simulink model "MagLevCtrl"  (R2025b)
settings: Solver=FixedStepDiscrete  StartTime=0.0  StopTime=Inf  FixedStep=Ts  RelTol=1e-3  EnableMultiTasking=on
undefined symbols (not defined in the file or in its folder): ctrl, DiscIntNeverNeededParam, enable, sens, X, Y
libraries: MagLevTbx_BaseLib x10, simulink x4
settings Model: ExtModeTrigDuration=2  Creator=riccardo  LastModifiedBy=riccardo
settings SolverCC: AutoInsertRateTranBlk=on
settings DataIOCC: ReturnWorkspaceOutputs=off
settings OptimizationCC: StrengthReduction=on  PassReuseOutputArgsAs=Individual arguments  ZeroExternalMemoryAtStartup=off  ZeroInternalMemoryAtStartup=off  MaxStackSize=64  OptimizeBlockOrder=speed  OptimizationPriority=Speed  OptimizationCustomize=off  MultiThreadedLoops=on  AutoScheduleForLoops=on  EfficientTunableParamExpr=on
settings DebuggingCC: ParameterTunabilityLossMsg=error
settings HardwareCC: ProdBitPerPointer=32.0  ProdBitPerSizeT=32.0  ProdBitPerPtrDiffT=32.0  ProdLargestAtomicInteger=Long  ProdLargestAtomicFloat=Double  ProdWordSize=32.0  ProdHWDeviceType=ARM Compatible->ARM Cortex
settings SFSimCC: MATLABDynamicMemAlloc=off
settings RTWCC: SystemTargetFile=ert.tlc  HardwareBoard=Teensy 4.1 (Arduino Compatible)  TemplateMakefile=ert_default_tmf  Toolchain=Arduino ARM M7  BuildConfiguration=Faster Runs  Description=Embedded Coder
settings CodeAppCC: ForceParamTrailComments=on  IgnoreCustomStorageClasses=off  OperatorAnnotations=on  SimulinkDataObjDesc=on  SFDataObjDesc=on  InsertBlockDesc=on
settings ERTTargetCC: ExtModeTransport=3.0  ExtModeStaticAlloc=on  ExtModeAutomaticAllocSize=off  ExtModeStaticAllocSize=65536.0  ExtModeMexFile=ext_xcp  ExtModeIntrfLevel=Level2 - Open  InlinedParameterPlacement=Hierarchical  RootIOFormat=Structure reference  TargetLangStandard=C99 (ISO)  SupportContinuousTime=on  SupportVariableSizeSignals=on

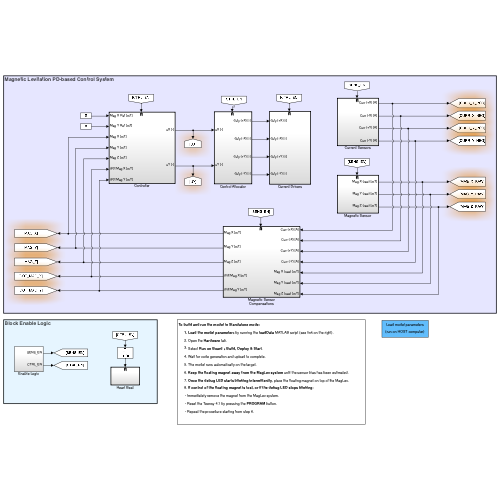
[thumbnail: Simulink's stored preview of the top-level diagram]
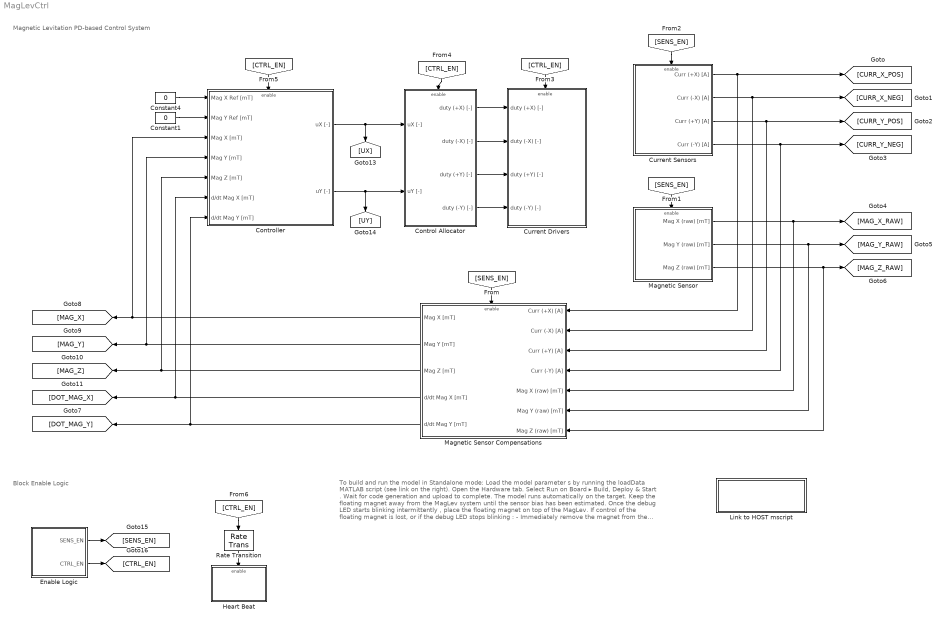
== system MagLevCtrl ==
  note: Block Enable Logic
  note: Magnetic Levitation PD-based Control System
  note: To build and run the model in Standalone mode:
      | Load the model parameter s by running the loadData MATLAB script (see link on the right).
      | Open the Hardware tab.
      | Select Run on Board ▸ Build, Deploy & Start .
      | Wait for code generation and upload to complete.
      | The model runs automatically on the target.
      | Keep the floating magnet away from the MagLev system until the sensor bias has been estimated.
      | Once the debug LED starts blinking intermittently , place the floating magnet on top of the MagLev.
      | If control of the floating magnet is lost, or if the debug LED stops blinking :
      | - Immediately remove the magnet from the MagLev system.
      | - Reset the Teensy 4.1 by pressing the PROGRAM button.
      | - Repeat the procedure starting from step 6.
  Constant1 : Constant  Value=0  OutDataTypeStr=single  SampleTime=ctrl.Ts
  Constant4 : Constant  Value=0  OutDataTypeStr=single  SampleTime=ctrl.Ts
  Control Allocator : Subsystem
  Controller : Subsystem
  Current Drivers : Subsystem
  Current Sensors : Subsystem
  Enable Logic : Subsystem
  Heart Beat : Subsystem
  Link to HOST mscript : Subsystem
      settings: OpenFcn=|
      | %  get toolbox base dir
      | info = MagLevTbx_Info();
      | 
      | %  path to HOST matlab script
      | mscriptpath = fullfile( ...
      | info.rootDir, ...
      | 'Examples', ...
      | 'Ctrl_Test', ...
      | 'Standalone', ...
      | 'loadData'  );
      | 
      | %  open script
      | edit( mscriptpath );
      | 
      | %  clear temp vars
      | clear info mscriptpath;
      mask Display:
      | disp(['Load model parameters\n\n' ...
      |     '(run on HOST computer)'])
  Magnetic Sensor : Subsystem
  Magnetic Sensor Compensations : Subsystem
  Rate Transition : RateTransition  OutPortSampleTime=enable.heartBeat_Ts
  wires:
  Current Sensors/1(Curr (+X) [A]) -> Magnetic Sensor Compensations/1(Curr (+X) [A]), [CURR_X_POS]
  Current Sensors/2(Curr (-X) [A]) -> Magnetic Sensor Compensations/2(Curr (-X) [A]), [CURR_X_NEG]
  Current Sensors/3(Curr (+Y) [A]) -> Magnetic Sensor Compensations/3(Curr (+Y) [A]), [CURR_Y_POS]
  Current Sensors/4(Curr (-Y) [A]) -> Magnetic Sensor Compensations/4(Curr (-Y) [A]), [CURR_Y_NEG]
  Magnetic Sensor/1(Mag X (raw) [mT]) -> Magnetic Sensor Compensations/5(Mag X (raw) [mT]), [MAG_X_RAW]
  Magnetic Sensor/2(Mag Y (raw) [mT]) -> Magnetic Sensor Compensations/6(Mag Y (raw) [mT]), [MAG_Y_RAW]
  Magnetic Sensor/3(Mag Z (raw) [mT]) -> Magnetic Sensor Compensations/7(Mag Z (raw) [mT]), [MAG_Z_RAW]
  Control Allocator/1(duty (+X) [-]) -> Current Drivers/1(duty (+X) [-])
  Control Allocator/2(duty (-X) [-]) -> Current Drivers/2(duty (-X) [-])
  Control Allocator/3(duty (+Y) [-]) -> Current Drivers/3(duty (+Y) [-])
  Control Allocator/4(duty (-Y) [-]) -> Current Drivers/4(duty (-Y) [-])
  Magnetic Sensor Compensations/2(Mag Y [mT]) -> [MAG_Y], Controller/4(Mag Y [mT])
  Magnetic Sensor Compensations/1(Mag X [mT]) -> [MAG_X], Controller/3(Mag X [mT])
  Constant4/1 -> Controller/1(Mag X Ref [mT])
  Constant1/1 -> Controller/2(Mag Y Ref [mT])
  Magnetic Sensor Compensations/4(d/dt Mag X [mT]) -> [DOT_MAG_X], Controller/6(d/dt Mag X [mT])
  Magnetic Sensor Compensations/5(d/dt Mag Y [mT]) -> [DOT_MAG_Y], Controller/7(d/dt Mag Y [mT])
  Magnetic Sensor Compensations/3(Mag Z [mT]) -> [MAG_Z], Controller/5(Mag Z [mT])
  [SENS_EN] -> Magnetic Sensor Compensations/Enable
  [SENS_EN] -> Magnetic Sensor/Enable
  [CTRL_EN] -> Control Allocator/Enable
  [CTRL_EN] -> Controller/Enable
  Enable Logic/1(SENS_EN) -> [SENS_EN]
  [SENS_EN] -> Current Sensors/Enable
  Enable Logic/2(CTRL_EN) -> [CTRL_EN]
  [CTRL_EN] -> Current Drivers/Enable
  Controller/1(uX [-]) -> Control Allocator/1(uX [-]), [UX]
  Controller/2(uY [-]) -> Control Allocator/2(uY [-]), [UY]
  [CTRL_EN] -> Rate Transition/1
  Rate Transition/1 -> Heart Beat/Enable

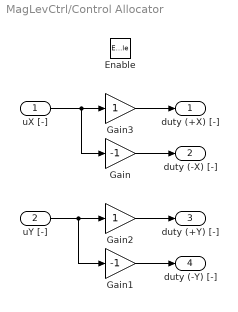
== system MagLevCtrl/Control Allocator ==
  uX [-] : Inport
  uY [-] : Inport  Port=2
  Enable : EnablePort
  Gain : Gain  Gain=-1
  Gain1 : Gain  Gain=-1
  Gain2 : Gain
  Gain3 : Gain
  duty (+X) [-] : Outport  OutputWhenDisabled=reset  InitialOutput=0
  duty (-X) [-] : Outport  Port=2  OutputWhenDisabled=reset  InitialOutput=0
  duty (+Y) [-] : Outport  Port=3  OutputWhenDisabled=reset  InitialOutput=0
  duty (-Y) [-] : Outport  Port=4  OutputWhenDisabled=reset  InitialOutput=0
  wires:
  uX [-]/1 -> Gain3/1, Gain/1
  Gain/1 -> duty (-X) [-]/1
  Gain1/1 -> duty (-Y) [-]/1
  uY [-]/1 -> Gain2/1, Gain1/1
  Gain2/1 -> duty (+Y) [-]/1
  Gain3/1 -> duty (+X) [-]/1

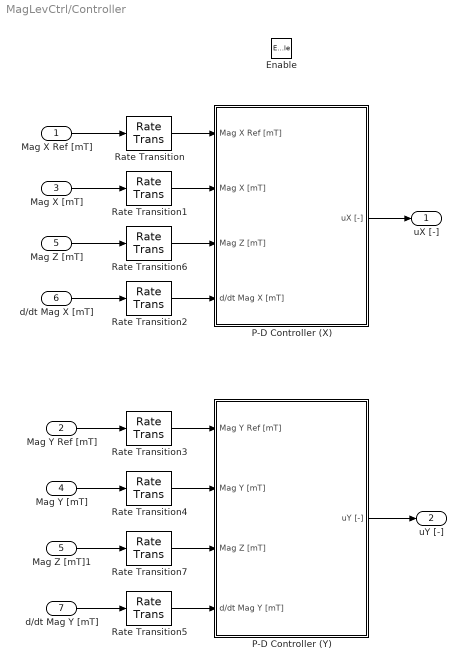
== system MagLevCtrl/Controller ==
  Mag X Ref [mT] : Inport
  Mag Y Ref [mT] : Inport  Port=2
  Mag X [mT] : Inport  Port=3
  Mag Y [mT] : Inport  Port=4
  Mag Z [mT] : Inport  Port=5
  d/dt Mag X [mT] : Inport  Port=6
  d/dt Mag Y [mT] : Inport  Port=7
  Enable : EnablePort
  Mag Z [mT]1 : InportShadow  Port=5
  P-D Controller (X) : Subsystem
  P-D Controller (Y) : Subsystem
  Rate Transition{,1..7} (8 alike) : RateTransition  OutPortSampleTime=ctrl.Ts
  uX [-] : Outport  OutputWhenDisabled=reset  InitialOutput=0
  uY [-] : Outport  Port=2  OutputWhenDisabled=reset  InitialOutput=0
  wires:
  d/dt Mag Y [mT]/1 -> Rate Transition5/1
  P-D Controller (Y)/1(uY [-]) -> uY [-]/1
  Mag Y Ref [mT]/1 -> Rate Transition3/1
  Mag X Ref [mT]/1 -> Rate Transition/1
  P-D Controller (X)/1(uX [-]) -> uX [-]/1
  Mag X [mT]/1 -> Rate Transition1/1
  Mag Y [mT]/1 -> Rate Transition4/1
  d/dt Mag X [mT]/1 -> Rate Transition2/1
  Rate Transition/1 -> P-D Controller (X)/1(Mag X Ref [mT])
  Rate Transition1/1 -> P-D Controller (X)/2(Mag X [mT])
  Rate Transition2/1 -> P-D Controller (X)/4(d/dt Mag X [mT])
  Rate Transition3/1 -> P-D Controller (Y)/1(Mag Y Ref [mT])
  Rate Transition4/1 -> P-D Controller (Y)/2(Mag Y [mT])
  Rate Transition5/1 -> P-D Controller (Y)/4(d/dt Mag Y [mT])
  Mag Z [mT]/1 -> Rate Transition6/1
  Rate Transition6/1 -> P-D Controller (X)/3(Mag Z [mT])
  Mag Z [mT]1/1 -> Rate Transition7/1
  Rate Transition7/1 -> P-D Controller (Y)/3(Mag Z [mT])

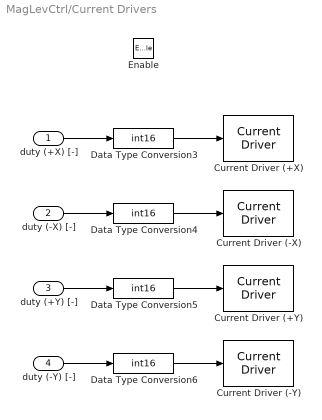
== system MagLevCtrl/Current Drivers ==
  duty (+X) [-] : Inport
  duty (-X) [-] : Inport  Port=2
  duty (+Y) [-] : Inport  Port=3
  duty (-Y) [-] : Inport  Port=4
  Enable : EnablePort
  Current Driver (+X) : MagLevTbx_BaseLib/Outputs/Current Driver  driverId=+X  sampleTime=ctrl.Ts  showEnablePort=off
      settings: SourceProductName=MagLev Toolbox
  Current Driver (+Y) : MagLevTbx_BaseLib/Outputs/Current Driver  driverId=+Y  sampleTime=ctrl.Ts  showEnablePort=off
      settings: SourceProductName=MagLev Toolbox
  Current Driver (-X) : MagLevTbx_BaseLib/Outputs/Current Driver  driverId=-X  sampleTime=ctrl.Ts  showEnablePort=off
      settings: SourceProductName=MagLev Toolbox
  Current Driver (-Y) : MagLevTbx_BaseLib/Outputs/Current Driver  driverId=-Y  sampleTime=ctrl.Ts  showEnablePort=off
      settings: SourceProductName=MagLev Toolbox
  Data Type Conversion{3..6} (4 alike) : DataTypeConversion  OutDataTypeStr=int16  SaturateOnIntegerOverflow=off  RndMeth=Floor
  wires:
  duty (+Y) [-]/1 -> Data Type Conversion5/1
  Data Type Conversion5/1 -> Current Driver (+Y)/1
  Data Type Conversion6/1 -> Current Driver (-Y)/1
  duty (-Y) [-]/1 -> Data Type Conversion6/1
  Data Type Conversion4/1 -> Current Driver (-X)/1
  duty (+X) [-]/1 -> Data Type Conversion3/1
  duty (-X) [-]/1 -> Data Type Conversion4/1
  Data Type Conversion3/1 -> Current Driver (+X)/1

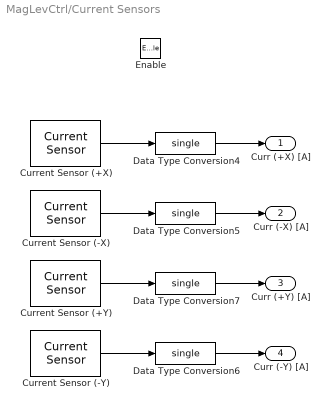
== system MagLevCtrl/Current Sensors ==
  Enable : EnablePort
  Current Sensor (+X) : MagLevTbx_BaseLib/Inputs/Current Sensor  sensorId=+X  sampleTime=sens.Ts  showEnablePort=off
      settings: SourceProductName=MagLev Toolbox
  Current Sensor (+Y) : MagLevTbx_BaseLib/Inputs/Current Sensor  sensorId=+Y  sampleTime=sens.Ts  showEnablePort=off
      settings: SourceProductName=MagLev Toolbox
  Current Sensor (-X) : MagLevTbx_BaseLib/Inputs/Current Sensor  sensorId=-X  sampleTime=sens.Ts  showEnablePort=off
      settings: SourceProductName=MagLev Toolbox
  Current Sensor (-Y) : MagLevTbx_BaseLib/Inputs/Current Sensor  sensorId=-Y  sampleTime=sens.Ts  showEnablePort=off
      settings: SourceProductName=MagLev Toolbox
  Data Type Conversion{4..7} (4 alike) : DataTypeConversion  OutDataTypeStr=single  SaturateOnIntegerOverflow=off  RndMeth=Floor
  Curr (+X) [A] : Outport
  Curr (-X) [A] : Outport  Port=2
  Curr (+Y) [A] : Outport  Port=3
  Curr (-Y) [A] : Outport  Port=4
  wires:
  Data Type Conversion5/1 -> Curr (-X) [A]/1
  Data Type Conversion4/1 -> Curr (+X) [A]/1
  Data Type Conversion7/1 -> Curr (+Y) [A]/1
  Data Type Conversion6/1 -> Curr (-Y) [A]/1
  Current Sensor (+X)/1 -> Data Type Conversion4/1
  Current Sensor (-X)/1 -> Data Type Conversion5/1
  Current Sensor (+Y)/1 -> Data Type Conversion7/1
  Current Sensor (-Y)/1 -> Data Type Conversion6/1

== system MagLevCtrl/Enable Logic ==
  Clock : Clock
  Interval Test : simulink/Logic and Bit Operations/Interval Test  IntervalClosedRight=on  uplimit=enable.ctrlTurnOffTime  IntervalClosedLeft=on  lowlimit=enable.ctrlTurnOnTime  OutDataTypeStr=boolean
  Interval Test1 : simulink/Logic and Bit Operations/Interval Test  IntervalClosedRight=on  uplimit=enable.sensTurnOffTime  IntervalClosedLeft=on  lowlimit=enable.sensTurnOnTime  OutDataTypeStr=boolean
  Rate Transition : RateTransition  OutPortSampleTime=enable.Ts
  Rate Transition1 : RateTransition  OutPortSampleTime=enable.Ts
  SENS_EN : Outport
  CTRL_EN : Outport  Port=2
  wires:
  Interval Test/1 -> Rate Transition/1
  Rate Transition/1 -> CTRL_EN/1
  Clock/1 -> Interval Test/1, Interval Test1/1
  Interval Test1/1 -> Rate Transition1/1
  Rate Transition1/1 -> SENS_EN/1

== system MagLevCtrl/Heart Beat ==
  Enable : EnablePort
  Data Type Conversion3 : DataTypeConversion  OutDataTypeStr=boolean  SaturateOnIntegerOverflow=off  RndMeth=Floor
  Repeating Sequence Stair : simulink/Sources/Repeating Sequence Stair  OutValues=[1 0].'  tsamp=enable.heartBeat_Ts  OutMin=[]  OutMax=[]  OutDataTypeStr=double  OutputDataTypeScalingMode=double  OutDataType=fixdt(0,8)  ConRadixGroup=Best Precision: Vector-wise  OutScaling=2^-12
  User LED : MagLevTbx_BaseLib/Outputs/User LED  sampleTime=-1  showEnablePort=off
      settings: SourceProductName=MagLev Toolbox
  wires:
  Repeating Sequence Stair/1 -> Data Type Conversion3/1
  Data Type Conversion3/1 -> User LED/1

== system MagLevCtrl/Link to HOST mscript ==

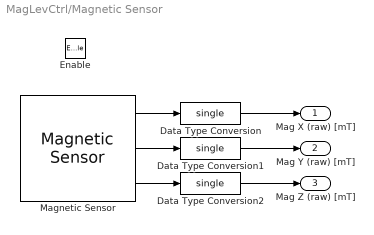
== system MagLevCtrl/Magnetic Sensor ==
  Enable : EnablePort
  Data Type Conversion : DataTypeConversion  OutDataTypeStr=single  SaturateOnIntegerOverflow=off  RndMeth=Floor
  Data Type Conversion1 : DataTypeConversion  OutDataTypeStr=single  SaturateOnIntegerOverflow=off  RndMeth=Floor
  Data Type Conversion2 : DataTypeConversion  OutDataTypeStr=single  SaturateOnIntegerOverflow=off  RndMeth=Floor
  Magnetic Sensor : MagLevTbx_BaseLib/Inputs/Magnetic Sensor  sensorId=Sensor 7  sampleTime=sens.Ts  showEnablePort=off
      settings: SourceProductName=MagLev Toolbox
  Mag X (raw) [mT] : Outport
  Mag Y (raw) [mT] : Outport  Port=2
  Mag Z (raw) [mT] : Outport  Port=3
  wires:
  Data Type Conversion1/1 -> Mag Y (raw) [mT]/1
  Data Type Conversion2/1 -> Mag Z (raw) [mT]/1
  Magnetic Sensor/2 -> Data Type Conversion1/1
  Data Type Conversion/1 -> Mag X (raw) [mT]/1
  Magnetic Sensor/1 -> Data Type Conversion/1
  Magnetic Sensor/3 -> Data Type Conversion2/1

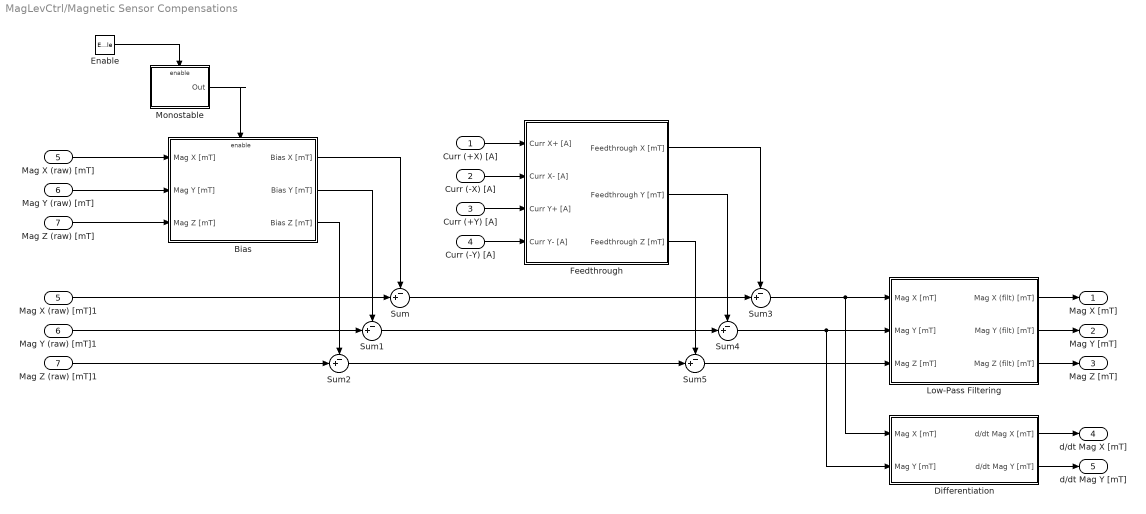
== system MagLevCtrl/Magnetic Sensor Compensations ==
  Curr (+X) [A] : Inport
  Curr (-X) [A] : Inport  Port=2
  Curr (+Y) [A] : Inport  Port=3
  Curr (-Y) [A] : Inport  Port=4
  Mag X (raw) [mT] : Inport  Port=5
  Mag Y (raw) [mT] : Inport  Port=6
  Mag Z (raw) [mT] : Inport  Port=7
  Enable : EnablePort  ShowOutputPort=on
  Bias : Subsystem
  Differentiation : Subsystem
  "Feedthrough " : Subsystem
  Low-Pass Filtering : Subsystem
  Mag X (raw) [mT]1 : InportShadow  Port=5
  Mag Y (raw) [mT]1 : InportShadow  Port=6
  Mag Z (raw) [mT]1 : InportShadow  Port=7
  Monostable : Subsystem  mask{Tp=enable.biasEvalTime}
      mask prompts: Tp "Pulse duration [s]"
  Sum{,1..5} (6 alike) : Sum  Inputs=-+|
  Mag X [mT] : Outport
  Mag Y [mT] : Outport  Port=2
  Mag Z [mT] : Outport  Port=3
  d/dt Mag X [mT] : Outport  Port=4
  d/dt Mag Y [mT] : Outport  Port=5
  wires:
  Bias/3(Bias Z [mT]) -> Sum2/1
  Bias/2(Bias Y [mT]) -> Sum1/1
  Mag Z (raw) [mT]/1 -> Bias/3(Mag Z [mT])
  Mag Y (raw) [mT]/1 -> Bias/2(Mag Y [mT])
  Mag X (raw) [mT]/1 -> Bias/1(Mag X [mT])
  Mag X (raw) [mT]1/1 -> Sum/2
  Sum/1 -> Sum3/2
  Mag Y (raw) [mT]1/1 -> Sum1/2
  Mag Z (raw) [mT]1/1 -> Sum2/2
  Bias/1(Bias X [mT]) -> Sum/1
  Curr (+X) [A]/1 -> "Feedthrough "/1(Curr X+ [A])
  Curr (-X) [A]/1 -> "Feedthrough "/2(Curr X- [A])
  Curr (+Y) [A]/1 -> "Feedthrough "/3(Curr Y+ [A])
  Curr (-Y) [A]/1 -> "Feedthrough "/4(Curr Y- [A])
  Sum2/1 -> Sum5/2
  "Feedthrough "/3(Feedthrough Z [mT]) -> Sum5/1
  "Feedthrough "/2(Feedthrough Y [mT]) -> Sum4/1
  "Feedthrough "/1(Feedthrough X [mT]) -> Sum3/1
  Sum1/1 -> Sum4/2
  Sum3/1 -> Differentiation/1(Mag X [mT]), Low-Pass Filtering/1(Mag X [mT])
  Sum4/1 -> Differentiation/2(Mag Y [mT]), Low-Pass Filtering/2(Mag Y [mT])
  Sum5/1 -> Low-Pass Filtering/3(Mag Z [mT])
  Low-Pass Filtering/1(Mag X (filt) [mT]) -> Mag X [mT]/1
  Low-Pass Filtering/2(Mag Y (filt) [mT]) -> Mag Y [mT]/1
  Low-Pass Filtering/3(Mag Z (filt) [mT]) -> Mag Z [mT]/1
  Monostable/1(Out) -> Bias/Enable
  Enable/1 -> Monostable/Enable
  Differentiation/1(d/dt Mag X [mT]) -> d/dt Mag X [mT]/1
  Differentiation/2(d/dt Mag Y [mT]) -> d/dt Mag Y [mT]/1

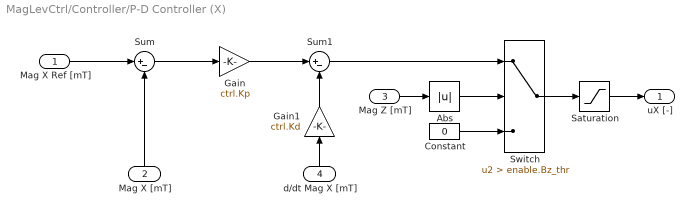
== system MagLevCtrl/Controller/P-D Controller (X) ==
  Mag X Ref [mT] : Inport
  Mag X [mT] : Inport  Port=2
  Mag Z [mT] : Inport  Port=3
  d/dt Mag X [mT] : Inport  Port=4
  Abs : Abs  SaturateOnIntegerOverflow=off
  Constant : Constant  Value=0  OutDataTypeStr=single
  Gain : Gain  Gain=ctrl.Kp
  Gain1 : Gain  Gain=ctrl.Kd
  Saturation : Saturate  UpperLimit=ctrl.outMax  LowerLimit=ctrl.outMin
  Sum : Sum  Inputs=|+-
  Sum1 : Sum  Inputs=|+-
  Switch : Switch  Criteria=u2 > Threshold  Threshold=enable.Bz_thr  SaturateOnIntegerOverflow=off  InputSameDT=off
  uX [-] : Outport  OutputWhenDisabled=reset  InitialOutput=0
  wires:
  Mag X Ref [mT]/1 -> Sum/1
  Sum/1 -> Gain/1
  Gain/1 -> Sum1/1
  Gain1/1 -> Sum1/2
  Mag X [mT]/1 -> Sum/2
  d/dt Mag X [mT]/1 -> Gain1/1
  Switch/1 -> Saturation/1
  Abs/1 -> Switch/2
  Constant/1 -> Switch/3
  Sum1/1 -> Switch/1
  Saturation/1 -> uX [-]/1
  Mag Z [mT]/1 -> Abs/1

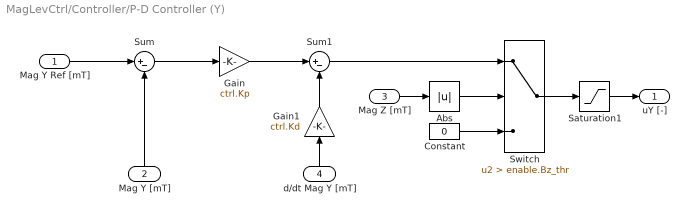
== system MagLevCtrl/Controller/P-D Controller (Y) ==
  Mag Y Ref [mT] : Inport
  Mag Y [mT] : Inport  Port=2
  Mag Z [mT] : Inport  Port=3
  d/dt Mag Y [mT] : Inport  Port=4
  Abs : Abs  SaturateOnIntegerOverflow=off
  Constant : Constant  Value=0  OutDataTypeStr=single
  Gain : Gain  Gain=ctrl.Kp
  Gain1 : Gain  Gain=ctrl.Kd
  Saturation1 : Saturate  UpperLimit=ctrl.outMax  LowerLimit=ctrl.outMin
  Sum : Sum  Inputs=|+-
  Sum1 : Sum  Inputs=|+-
  Switch : Switch  Criteria=u2 > Threshold  Threshold=enable.Bz_thr  SaturateOnIntegerOverflow=off  InputSameDT=off
  uY [-] : Outport  OutputWhenDisabled=reset  InitialOutput=0
  wires:
  d/dt Mag Y [mT]/1 -> Gain1/1
  Mag Y [mT]/1 -> Sum/2
  Gain1/1 -> Sum1/2
  Gain/1 -> Sum1/1
  Sum/1 -> Gain/1
  Mag Y Ref [mT]/1 -> Sum/1
  Saturation1/1 -> uY [-]/1
  Mag Z [mT]/1 -> Abs/1
  Switch/1 -> Saturation1/1
  Abs/1 -> Switch/2
  Sum1/1 -> Switch/1
  Constant/1 -> Switch/3

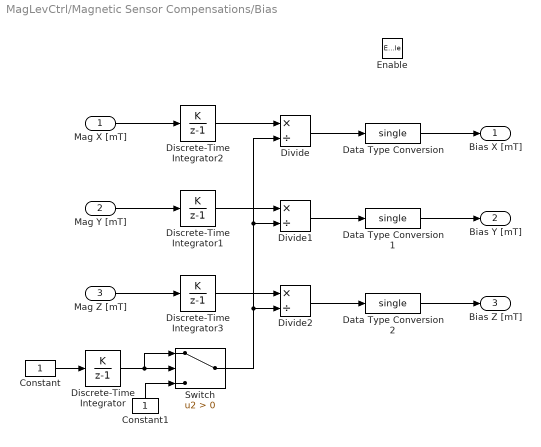
== system MagLevCtrl/Magnetic Sensor Compensations/Bias ==
  Mag X [mT] : Inport
  Mag Y [mT] : Inport  Port=2
  Mag Z [mT] : Inport  Port=3
  Enable : EnablePort  StatesWhenEnabling=reset
  Constant : Constant
  Constant1 : Constant
  Data Type Conversion : DataTypeConversion  OutDataTypeStr=single  SaturateOnIntegerOverflow=off  RndMeth=Floor
  Data Type Conversion1 : DataTypeConversion  OutDataTypeStr=single  SaturateOnIntegerOverflow=off  RndMeth=Floor
  Data Type Conversion2 : DataTypeConversion  OutDataTypeStr=single  SaturateOnIntegerOverflow=off  RndMeth=Floor
  Discrete-Time Integrator{,1..3} (4 alike) : DiscreteIntegrator  IntegratorMethod=Accumulation: Forward Euler  SampleTime=-1  ICPrevOutput=DiscIntNeverNeededParam  ICPrevScaledInput=DiscIntNeverNeededParam
  Divide : Product  Inputs=*/
  Divide1 : Product  Inputs=*/
  Divide2 : Product  Inputs=*/
  Switch : Switch  Criteria=u2 > Threshold  SaturateOnIntegerOverflow=off  InputSameDT=off
  Bias X [mT] : Outport  VectorParamsAs1DForOutWhenUnconnected=off
  Bias Y [mT] : Outport  Port=2  VectorParamsAs1DForOutWhenUnconnected=off
  Bias Z [mT] : Outport  Port=3  VectorParamsAs1DForOutWhenUnconnected=off
  wires:
  Discrete-Time Integrator1/1 -> Divide1/1
  Constant/1 -> Discrete-Time Integrator/1
  Discrete-Time Integrator2/1 -> Divide/1
  Mag X [mT]/1 -> Discrete-Time Integrator2/1
  Mag Z [mT]/1 -> Discrete-Time Integrator3/1
  Mag Y [mT]/1 -> Discrete-Time Integrator1/1
  Discrete-Time Integrator3/1 -> Divide2/1
  Divide/1 -> Data Type Conversion/1
  Divide1/1 -> Data Type Conversion1/1
  Divide2/1 -> Data Type Conversion2/1
  Discrete-Time Integrator/1 -> Switch/1, Switch/2
  Switch/1 -> Divide2/2, Divide/2, Divide1/2
  Constant1/1 -> Switch/3
  Data Type Conversion2/1 -> Bias Z [mT]/1
  Data Type Conversion1/1 -> Bias Y [mT]/1
  Data Type Conversion/1 -> Bias X [mT]/1

== system MagLevCtrl/Magnetic Sensor Compensations/Differentiation ==
  Mag X [mT] : Inport
  Mag Y [mT] : Inport  Port=2
  Discrete Transfer Fcn : DiscreteTransferFcn  Numerator=sens.hpf.num  Denominator=sens.hpf.den
  Discrete Transfer Fcn1 : DiscreteTransferFcn  Numerator=sens.hpf.num  Denominator=sens.hpf.den
  d/dt Mag X [mT] : Outport
  d/dt Mag Y [mT] : Outport  Port=2
  wires:
  Discrete Transfer Fcn/1 -> d/dt Mag X [mT]/1
  Discrete Transfer Fcn1/1 -> d/dt Mag Y [mT]/1
  Mag Y [mT]/1 -> Discrete Transfer Fcn1/1
  Mag X [mT]/1 -> Discrete Transfer Fcn/1

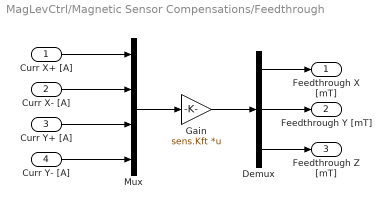
== system MagLevCtrl/Magnetic Sensor Compensations/Feedthrough  ==
  Curr X+ [A] : Inport
  Curr X- [A] : Inport  Port=2
  Curr Y+ [A] : Inport  Port=3
  Curr Y- [A] : Inport  Port=4
  Demux : Demux  Outputs=3
  Gain : Gain  Gain=sens.Kft  Multiplication=Matrix(K*u) (u vector)
  Mux : Mux
  Feedthrough X [mT] : Outport
  Feedthrough Y [mT] : Outport  Port=2
  Feedthrough Z [mT] : Outport  Port=3
  wires:
  Curr X+ [A]/1 -> Mux/1
  Demux/2 -> Feedthrough Y [mT]/1
  Curr Y+ [A]/1 -> Mux/3
  Demux/3 -> Feedthrough Z [mT]/1
  Curr X- [A]/1 -> Mux/2
  Curr Y- [A]/1 -> Mux/4
  Gain/1 -> Demux/1
  Demux/1 -> Feedthrough X [mT]/1
  Mux/1 -> Gain/1

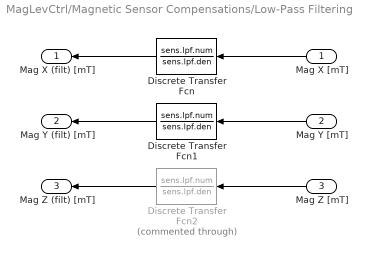
== system MagLevCtrl/Magnetic Sensor Compensations/Low-Pass Filtering ==
  Mag X [mT] : Inport
  Mag Y [mT] : Inport  Port=2
  Mag Z [mT] : Inport  Port=3
  Discrete Transfer Fcn : DiscreteTransferFcn  Numerator=sens.lpf.num  Denominator=sens.lpf.den
  Discrete Transfer Fcn1 : DiscreteTransferFcn  Numerator=sens.lpf.num  Denominator=sens.lpf.den
  Discrete Transfer Fcn2 : DiscreteTransferFcn  Commented=through  Numerator=sens.lpf.num  Denominator=sens.lpf.den
  Mag X (filt) [mT] : Outport
  Mag Y (filt) [mT] : Outport  Port=2
  Mag Z (filt) [mT] : Outport  Port=3
  wires:
  Discrete Transfer Fcn1/1 -> Mag Y (filt) [mT]/1
  Mag Y [mT]/1 -> Discrete Transfer Fcn1/1
  Mag X [mT]/1 -> Discrete Transfer Fcn/1
  Discrete Transfer Fcn/1 -> Mag X (filt) [mT]/1
  Mag Z [mT]/1 -> Discrete Transfer Fcn2/1
  Discrete Transfer Fcn2/1 -> Mag Z (filt) [mT]/1

== system MagLevCtrl/Magnetic Sensor Compensations/Monostable ==
  Enable : EnablePort  StatesWhenEnabling=reset
  Compare To Constant : simulink/Logic and Bit Operations/Compare To Constant  relop=<  const=Tp  OutDataTypeStr=boolean
  Constant1 : Constant
  Discrete-Time Integrator : DiscreteIntegrator  SampleTime=-1  LimitOutput=on  UpperSaturationLimit=Tp  LowerSaturationLimit=0  ICPrevOutput=DiscIntNeverNeededParam  ICPrevScaledInput=DiscIntNeverNeededParam
  Out : Outport  VectorParamsAs1DForOutWhenUnconnected=off
  wires:
  Discrete-Time Integrator/1 -> Compare To Constant/1
  Constant1/1 -> Discrete-Time Integrator/1
  Compare To Constant/1 -> Out/1
